simulink model "simulador2017b_v1"  (R2017b)
settings: Solver=FixedStepAuto  StartTime=0.0  StopTime=10  FixedStep=ST  RelTol=1e-3
undefined symbols (not defined in the file or in its folder): b, c_bar, CD_deltae, CDp, CDq, CL0, Cl0, CL_alpha, Cl_beta, Cl_da, CL_deltae, Cl_dr, Cl_p, Cl_r, CLq, Cm0, Cm_alpha, Cm_de, Cm_df, Cm_q, Cn0, Cn_beta, Cn_da, Cn_dr, Cn_p, Cn_r, Cx_df, Cx_dr, Cy0, Cy_beta, Cy_da, Cy_dr, Cy_p, Cy_r, Cz_df, delta_max, Earth, F, i0, k1, k2, KQ, Kv, Light, M, mass, maxRPM, MIL, N, R, ST, T, V, Vmax, Vw_unif, WGS84
libraries: aerolibwind2 x3, aerolibtransform2 x2, aerolibasang x2, aerolibanimutils x1, aerolibfltsims x1, simulink_extras x1, aerolibatmos2 x1, shared6dof x1, aerolibadyn x1
(part 1 of 2)
settings Model: Creator=rablanco.ext  LastModifiedBy=CC
settings SolverCC: ZeroCrossAlgorithm=Adaptive
settings DebuggingCC: AlgebraicLoopMsg=none

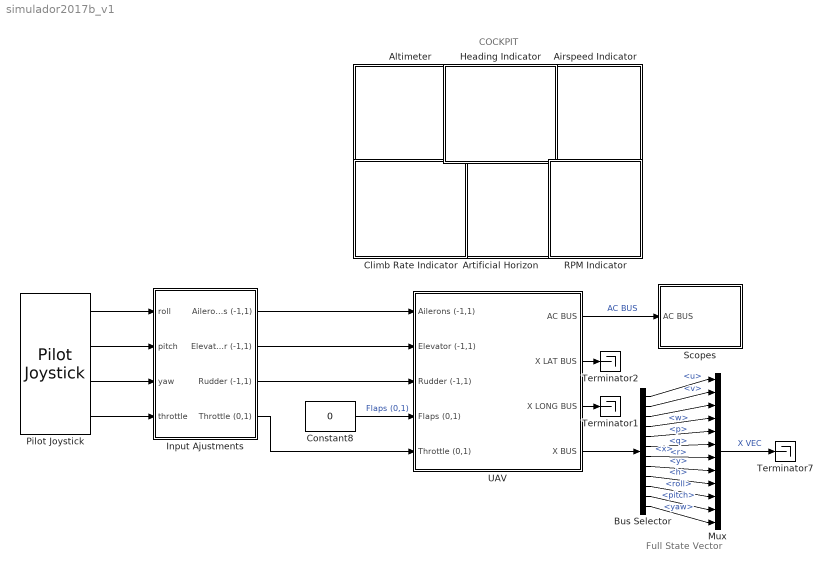
== system simulador2017b_v1 ==
  note: COCKPIT
  note: Full State Vector
  Airspeed Indicator : Subsystem  DialogController=aeroblksHMICreateDDGDialog  IsWebBlock=on  mask(MWDashboardBlock){webBlockId=0719782b-36e5-44f5-ad02-04d1cd166071, webBlockType=airspeedindicator, ShowInLibBrowser=on, ShowInitialText=on, HMISrcModelName=simulador2017b_v1}
      mask prompts: webBlockId "WebBlock Id"; webBlockType "WebBlock Type"; HMISrcModelName "Source Model"
      mask help: Display aircraft airspeed in knots.
      mask Help: asbhmihelp('airspeedindicator')
      mask Display:
      | if strcmp(get_param(bdroot(gcb),'BlockDiagramType'), 'library')
      |  image([(matlabroot) '/toolbox/aeroblks/aeroblks/hmi/icons/AirspeedIndicatorIcon.svg'])
      | end
  Altimeter : Subsystem  DialogController=aeroblksHMICreateDDGDialog  IsWebBlock=on  mask(MWDashboardBlock){webBlockId=d9dc4979-4f2a-46e8-a381-7c2968eac84c, webBlockType=altimeter, ShowInLibBrowser=on, ShowInitialText=on, HMISrcModelName=simulador2017b_v1}
      mask prompts: webBlockId "WebBlock Id"; webBlockType "WebBlock Type"; HMISrcModelName "Source Model"
      mask help: Display aircraft altitude in feet.
      mask Help: asbhmihelp('altimeter')
      mask Display:
      | if strcmp(get_param(bdroot(gcb),'BlockDiagramType'), 'library')
      |  image([(matlabroot) '/toolbox/aeroblks/aeroblks/hmi/icons/AltimeterIcon.svg'])
      | end
  Artificial Horizon : Subsystem  DialogController=aeroblksHMICreateDDGDialog  IsWebBlock=on  mask(MWDashboardBlock){webBlockId=07832adf-b17d-4d9e-ad18-10cd735fd072, webBlockType=artificialhorizon, ShowInLibBrowser=on, ShowInitialText=on, HMISrcModelName=simulador2017b_v1}
      mask prompts: webBlockId "WebBlock Id"; webBlockType "WebBlock Type"; HMISrcModelName "Source Model"
      mask help: Display aircraft attitude relative to horizon. The two signal input vector contains roll and pitch.
      mask Help: asbhmihelp('artificialhorizon')
      mask Display:
      | if strcmp(get_param(bdroot(gcb),'BlockDiagramType'), 'library')
      |  image([(matlabroot) '/toolbox/aeroblks/aeroblks/hmi/icons/ArtificialHorizonIcon.svg'])
      | end
  Bus Selector : BusSelector  OutputSignals=u,v,w,p,q,r,x,y,h,roll,pitch,yaw
  Climb Rate Indicator : Subsystem  DialogController=aeroblksHMICreateDDGDialog  IsWebBlock=on  mask(MWDashboardBlock){webBlockId=6f82ebd9-12ab-4ae3-b879-fc3c75439e10, webBlockType=climbindicator, ShowInLibBrowser=on, ShowInitialText=on, HMISrcModelName=simulador2017b_v1}
      mask prompts: webBlockId "WebBlock Id"; webBlockType "WebBlock Type"; HMISrcModelName "Source Model"
      mask help: Display aircraft climb rate in ft/min.
      mask Help: asbhmihelp('climbindicator')
      mask Display:
      | if strcmp(get_param(bdroot(gcb),'BlockDiagramType'), 'library')
      |  image([(matlabroot) '/toolbox/aeroblks/aeroblks/hmi/icons/ClimbIndicatorIcon.svg'])
      | end
  Constant8 : Constant  Value=0
  Heading Indicator : Subsystem  DialogController=aeroblksHMICreateDDGDialog  IsWebBlock=on  mask(MWDashboardBlock){webBlockId=75353ccd-7314-467c-8fad-26cd782088f3, webBlockType=headingindicator, ShowInLibBrowser=on, ShowInitialText=on, HMISrcModelName=simulador2017b_v1}
      mask prompts: webBlockId "WebBlock Id"; webBlockType "WebBlock Type"; HMISrcModelName "Source Model"
      mask help: Display aircraft heading with respect to North in degrees.
      mask Help: asbhmihelp('headingindicator')
      mask Display:
      | if strcmp(get_param(bdroot(gcb),'BlockDiagramType'), 'library')
      |  image([(matlabroot) '/toolbox/aeroblks/aeroblks/hmi/icons/HeadingIndicatorIcon.svg'])
      | end
  Input Ajustments : Subsystem
  Mux : Mux  Inputs=12
  "Pilot Joystick " : aerolibanimutils/Pilot Joystick  JoystickID=Joystick1  OutputConfiguration=FourAxis  SampleTime=ST
  RPM Indicator : Subsystem  DialogController=aeroblksHMICreateDDGDialog  IsWebBlock=on  mask(MWDashboardBlock){webBlockId=8c376309-98f9-4b67-9096-3662e58f3d70, webBlockType=rpmindicator, ShowInLibBrowser=on, ShowInitialText=on, HMISrcModelName=simulador2017b_v1}
      mask prompts: webBlockId "WebBlock Id"; webBlockType "WebBlock Type"; HMISrcModelName "Source Model"
      mask help: Display engine revolutions per minute (RPM).
      mask Help: asbhmihelp('rpmindicator')
      mask Display:
      | if strcmp(get_param(bdroot(gcb),'BlockDiagramType'), 'library')
      |  image([(matlabroot) '/toolbox/aeroblks/aeroblks/hmi/icons/RPMIndicatorIcon.svg'])
      | end
  Scopes : Subsystem
  Terminator1 : Terminator
  Terminator2 : Terminator
  Terminator7 : Terminator
  UAV : Subsystem  InitFcn=run('..\config_model.m')  StopFcn=|  mask{eulerInit=[0.0014,-0.023,0], ratesInit=[0.1729,0,-0.0277], VbInit=[53.287,-0.958,-1.1917], XeInit=[0 0 -100]}
      | save simulationData Va beta alpha p_meas q_meas r_meas rho deltaa deltae deltar deltat accX accY accZ;
      | save fullStateData time u v w p q r x y z phi theta psi;
      | aileronValMatrix = [time,ailerons_val];
      | elevatorValMatrix = [time,elevator_val];
      | rudderValMatrix = [time,rudder_val];
      | throttleValMatrix = [time,throttle_val];
      mask DialogControl DescGroupVar Prompt: Fixed-Wing UAV Model - V3 - Simplified Version
      mask DialogControl DescTextVar Prompt: This version of the model uses a simplified propulsive model based on the Momentum Theory (Froude Ideal Theory or Disk Actuator Theory) and a simplified polar curve that consists of a linear relationship between the drag coefficient CD and the AOA.
      mask DialogControl Control2 Prompt: INITIAL CONDITIONS for the state integrators: X0.
      mask DialogControl Control4 Prompt: Euler Angles
      mask DialogControl Control4_copy_copy Prompt: Angular Rates - Body Axis
      mask DialogControl Control4_copy Prompt: Ground/Inertial Velocity - Body Axis
      mask DialogControl Control4_copy_copy_copy Prompt: Position (Flat-Earth Model) - NED Axis
  wires:
  UAV/4(X BUS) -> Bus Selector/1
  UAV/2(X LAT BUS) -> Terminator2/1
  UAV/3(X LONG BUS) -> Terminator1/1
  Bus Selector/3 -> Mux/3  "<w>"
  Bus Selector/4 -> Mux/4  "<p>"
  Bus Selector/5 -> Mux/5  "<q>"
  Bus Selector/6 -> Mux/6  "<r>"
  Bus Selector/9 -> Mux/9  "<h>"
  Bus Selector/1 -> Mux/1  "<u>"
  Bus Selector/2 -> Mux/2  "<v>"
  Mux/1 -> Terminator7/1  "X VEC"
  Bus Selector/10 -> Mux/10  "<roll>"
  Bus Selector/11 -> Mux/11  "<pitch>"
  Bus Selector/12 -> Mux/12  "<yaw>"
  Bus Selector/8 -> Mux/8  "<y>"
  Bus Selector/7 -> Mux/7  "<x>"
  UAV/1(AC BUS) -> Scopes/1(AC BUS)  "AC BUS"
  Input Ajustments/4(Throttle (0,1)) -> UAV/5(Throttle (0,1))
  "Pilot Joystick "/1 -> Input Ajustments/1(roll)
  Input Ajustments/3(Rudder (-1,1)) -> UAV/3(Rudder (-1,1))
  "Pilot Joystick "/2 -> Input Ajustments/2(pitch)
  "Pilot Joystick "/3 -> Input Ajustments/3(yaw)
  Input Ajustments/1(Ailerons (-1,1)) -> UAV/1(Ailerons (-1,1))
  Constant8/1 -> UAV/4(Flaps (0,1))  "Flaps (0,1)"
  Input Ajustments/2(Elevator (-1,1)) -> UAV/2(Elevator (-1,1))
  "Pilot Joystick "/4 -> Input Ajustments/4(throttle)

== system simulador2017b_v1/Airspeed Indicator ==

== system simulador2017b_v1/Altimeter ==

== system simulador2017b_v1/Artificial Horizon ==

== system simulador2017b_v1/Climb Rate Indicator ==

== system simulador2017b_v1/Heading Indicator ==

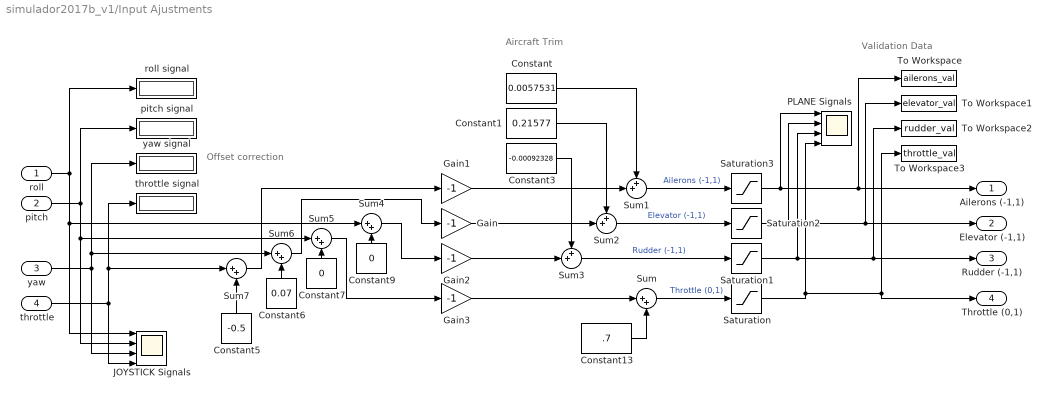
== system simulador2017b_v1/Input Ajustments ==
  note: Validation Data
  note: Aircraft Trim
  note: Offset correction
  roll : Inport
  pitch : Inport  Port=2
  yaw : Inport  Port=3
  throttle : Inport  Port=4
  Constant : Constant  Value=0.0057531
  Constant1 : Constant  Value=0.21577
  Constant13 : Constant  Value=.7
  Constant3 : Constant  Value=-0.00092328
  Constant5 : Constant  Value=-0.5
  Constant6 : Constant  Value=0.07
  Constant7 : Constant  Value=0
  Constant9 : Constant  Value=0
  Gain{,1..3} (4 alike) : Gain  Gain=-1
  "JOYSTICK Signals " : Scope  NumInputPorts=4
  "PLANE Signals " : Scope  NumInputPorts=4
  Saturation : Saturate  UpperLimit=1  LowerLimit=0
  Saturation1 : Saturate  UpperLimit=1  LowerLimit=-1
  Saturation2 : Saturate  UpperLimit=1  LowerLimit=-1
  Saturation3 : Saturate  UpperLimit=1  LowerLimit=-1
  Sum{,4..7} (5 alike) : Sum  Inputs=|++
  Sum1 : Sum  Inputs=++|
  Sum2 : Sum  Inputs=++|
  Sum3 : Sum  Inputs=++|
  To Workspace : ToWorkspace  VariableName=ailerons_val  SampleTime=-1
  To Workspace1 : ToWorkspace  VariableName=elevator_val  SampleTime=-1
  To Workspace2 : ToWorkspace  VariableName=rudder_val  SampleTime=-1
  To Workspace3 : ToWorkspace  VariableName=throttle_val  SampleTime=-1
  pitch signal : Display
  roll signal : Display
  throttle signal : Display
  yaw signal : Display
  Ailerons (-1,1) : Outport
  Elevator (-1,1) : Outport  Port=2
  Rudder (-1,1) : Outport  Port=3
  Throttle (0,1) : Outport  Port=4
  wires:
  pitch/1 -> "JOYSTICK Signals "/2, Sum5/1, pitch signal/1
  Constant1/1 -> Sum2/1
  throttle/1 -> Sum7/1, throttle signal/1, "JOYSTICK Signals "/4
  Sum/1 -> Saturation/1  "Throttle (0,1)"
  Constant/1 -> Sum1/1
  Constant7/1 -> Sum5/2
  Sum2/1 -> Saturation2/1  "Elevator (-1,1)"
  Gain2/1 -> Sum3/2
  roll/1 -> roll signal/1, "JOYSTICK Signals "/1, Sum4/1
  Sum4/1 -> Gain2/1
  Sum1/1 -> Saturation3/1  "Ailerons (-1,1)"
  Constant5/1 -> Sum7/2
  Gain1/1 -> Sum1/2
  Sum6/1 -> Gain/1
  Constant13/1 -> Sum/2
  Constant3/1 -> Sum3/1
  Sum3/1 -> Saturation1/1  "Rudder (-1,1)"
  Gain3/1 -> Sum/1
  yaw/1 -> yaw signal/1, Sum6/1, "JOYSTICK Signals "/3
  Sum7/1 -> Gain1/1
  Constant6/1 -> Sum6/2
  Constant9/1 -> Sum4/2
  Sum5/1 -> Gain3/1
  Gain/1 -> Sum2/2
  Saturation/1 -> "PLANE Signals "/4, Throttle (0,1)/1, To Workspace3/1
  Saturation1/1 -> "PLANE Signals "/3, Rudder (-1,1)/1, To Workspace2/1
  Saturation2/1 -> "PLANE Signals "/2, To Workspace1/1, Elevator (-1,1)/1
  Saturation3/1 -> "PLANE Signals "/1, To Workspace/1, Ailerons (-1,1)/1

== system simulador2017b_v1/RPM Indicator ==

== system simulador2017b_v1/Scopes ==
  AC BUS : Inport
  Attitude Scope : Scope  NumInputPorts=3
  Constant : Constant  Value=0
  Control Scope : Scope  NumInputPorts=5
  Demux : Demux  Outputs=2
  Flat Earth to LLA : aerolibtransform2/Flat Earth to LLA  units=Metric (MKS)  ptype=Earth (WGS84)  F=1/298.257223563  R=6378137  LL0=LatLong0  psi=0
  FlightGear Preconfigured 6DoF Animation : aerolibfltsims/FlightGear Preconfigured 6DoF Animation  xFlightGearVersion=v2017.1  DestinationIpAddress=127.0.0.1  DestinationPort=5502  SampleTime=0.01
      settings: SourceProductName=Aerospace Blockset
  Gain : Gain  Gain=-1
  Lateral Dynamics : Scope
  Longitudinal Dynamics : Scope
  Mux : Mux  Inputs=2
  Mux1 : Mux  Inputs=2
  Mux2 : Mux  Inputs=2
  Position Scope : Scope  NumInputPorts=3
  Propulsion Scope : Scope  NumInputPorts=3
  Selector : Selector  InputPortWidth=3  IndexOptions=Index vector (dialog)  Indices=[3]  OutputSizes=1
  Terminator : Terminator
  Visualization BOX : Subsystem
  wires:
  Visualization BOX/15(u (kph)) -> Propulsion Scope/2
  Visualization BOX/13(Throttle (%)) -> Control Scope/5
  Visualization BOX/8(Height_m) -> Position Scope/3
  Visualization BOX/11(Ailerons (deg)) -> Control Scope/3
  Visualization BOX/3(roll_deg) -> Attitude Scope/1
  AC BUS/1 -> Visualization BOX/1("AC BUS ")
  Visualization BOX/7(East_km) -> Position Scope/2
  Visualization BOX/9(Elevator (deg)) -> Control Scope/1
  Visualization BOX/10(Rudder (deg)) -> Control Scope/2
  Visualization BOX/14(<Thrust>) -> Propulsion Scope/1
  Visualization BOX/16(<RPM>) -> Propulsion Scope/3
  Visualization BOX/12(flaps (deg)) -> Control Scope/4
  Visualization BOX/4(pitch_deg) -> Attitude Scope/2
  Visualization BOX/6(North_km) -> Position Scope/1
  Visualization BOX/5(yaw_deg) -> Attitude Scope/3
  Visualization BOX/17(Longitudinal BUS) -> Longitudinal Dynamics/1
  Visualization BOX/18(Lateral BUS) -> Lateral Dynamics/1
  Mux2/1 -> Mux1/1
  Demux/2 -> Mux2/1
  Demux/1 -> Mux2/2
  Constant/1 -> Flat Earth to LLA/2
  Mux1/1 -> Mux/1
  Visualization BOX/1(Xe) -> Selector/1, Flat Earth to LLA/1
  Visualization BOX/2(<phi theta psi>) -> Mux/2
  Gain/1 -> Mux1/2
  Selector/1 -> Gain/1
  Mux/1 -> FlightGear Preconfigured 6DoF Animation/1
  Flat Earth to LLA/1 -> Demux/1
  Flat Earth to LLA/2 -> Terminator/1

== system simulador2017b_v1/UAV ==
  Ailerons (-1,1) : Inport
  Elevator (-1,1) : Inport  Port=2
  Rudder (-1,1) : Inport  Port=3
  Flaps (0,1) : Inport  Port=4
  Throttle (0,1) : Inport  Port=5
  AC State Creator : Subsystem
  Control BUS Creator : Subsystem
  Environment Model : Subsystem
  Flight Data Recorder (FDR) : Subsystem
  "Platform " : Subsystem
  AC BUS : Outport
  X LAT BUS : Outport  Port=2
  X LONG BUS : Outport  Port=3
  X BUS : Outport  Port=4
  wires:
  Environment Model/1(Environment BUS (ENV BUS)) -> "Platform "/1(ENV BUS)
  Control BUS Creator/1(Control BUS (CTRL BUS)) -> "Platform "/2(CTRL BUS)
  Elevator (-1,1)/1 -> Control BUS Creator/2(Elevator Command (-1,1))
  Flaps (0,1)/1 -> Control BUS Creator/4(Flaps Command (0,1))
  Rudder (-1,1)/1 -> Control BUS Creator/3(Rudder Command (-1,1))
  Ailerons (-1,1)/1 -> Control BUS Creator/1(Ailerons Command (-1,1))
  Throttle (0,1)/1 -> Control BUS Creator/5("Throttle Command (0,1) ")
  "Platform "/1(AC BUS) -> Flight Data Recorder (FDR)/1(AC BUS), Environment Model/1(AC BUS), AC BUS/1, AC State Creator/1(AC BUS)
  AC State Creator/1(X BUS) -> X BUS/1
  AC State Creator/2(X LONG BUS) -> X LONG BUS/1
  AC State Creator/3(X LAT BUS) -> X LAT BUS/1

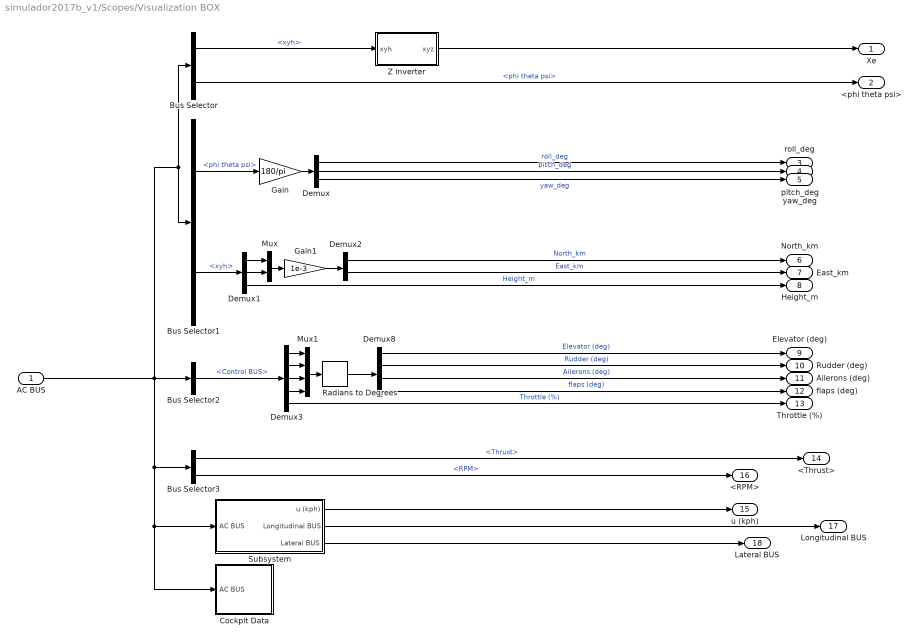
== system simulador2017b_v1/Scopes/Visualization BOX ==
  "AC BUS " : Inport
  Bus Selector : BusSelector  OutputSignals=xyh,phi theta psi
  Bus Selector1 : BusSelector  OutputSignals=phi theta psi,xyh
  Bus Selector2 : BusSelector  OutputSignals=Control BUS
  Bus Selector3 : BusSelector  OutputSignals=Propulsion Data BUS.Thrust,Propulsion Data BUS.RPM
  Cockpit Data : Subsystem
  Demux : Demux  Outputs=3
  Demux1 : Demux  Outputs=3
  Demux2 : Demux  Outputs=2
  Demux3 : Demux  Outputs=5
  Demux8 : Demux
  Gain : Gain  Gain=180/pi
  Gain1 : Gain  Gain=1e-3
  Mux : Mux  Inputs=2
  Mux1 : Mux
  Radians to Degrees : simulink_extras/Transformations/Radians to Degrees
  Subsystem : Subsystem
  Z inverter : Subsystem
  Xe : Outport
  <phi theta psi> : Outport  Port=2
  roll_deg : Outport  Port=3
  pitch_deg : Outport  Port=4
  yaw_deg : Outport  Port=5
  North_km : Outport  Port=6
  East_km : Outport  Port=7
  Height_m : Outport  Port=8
  Elevator (deg) : Outport  Port=9
  Rudder (deg) : Outport  Port=10
  Ailerons (deg) : Outport  Port=11
  flaps (deg) : Outport  Port=12
  Throttle (%) : Outport  Port=13
  <Thrust> : Outport  Port=14
  u (kph) : Outport  Port=15
  <RPM> : Outport  Port=16
  Longitudinal BUS : Outport  Port=17
  Lateral BUS : Outport  Port=18
  wires:
  Subsystem/2(Longitudinal BUS) -> Longitudinal BUS/1
  Subsystem/3(Lateral BUS) -> Lateral BUS/1
  Subsystem/1(u (kph)) -> u (kph)/1
  Bus Selector1/2 -> Demux1/1  "<xyh>"
  Demux1/3 -> Height_m/1  "Height_m"
  Demux/3 -> yaw_deg/1  "yaw_deg"
  Gain/1 -> Demux/1
  Demux/1 -> roll_deg/1  "roll_deg"
  Demux1/2 -> Mux/2
  Bus Selector1/1 -> Gain/1  "<phi theta psi>"
  Demux2/2 -> East_km/1  "East_km"
  Bus Selector2/1 -> Demux3/1  "<Control BUS>"
  Gain1/1 -> Demux2/1
  Bus Selector/2 -> <phi theta psi>/1  "<phi theta psi>"
  Bus Selector/1 -> Z inverter/1(xyh)  "<xyh>"
  Demux1/1 -> Mux/1
  "AC BUS "/1 -> Bus Selector3/1, Subsystem/1(AC BUS), Cockpit Data/1(AC BUS), Bus Selector2/1, Bus Selector/1, Bus Selector1/1
  Demux2/1 -> North_km/1  "North_km"
  Demux/2 -> pitch_deg/1  "pitch_deg"
  Mux/1 -> Gain1/1
  Demux3/4 -> Mux1/4
  Mux1/1 -> Radians to Degrees/1
  Demux3/5 -> Throttle (%)/1  "Throttle (%)"
  Bus Selector3/1 -> <Thrust>/1  "<Thrust>"
  Bus Selector3/2 -> <RPM>/1  "<RPM>"
  Radians to Degrees/1 -> Demux8/1
  Demux3/3 -> Mux1/3
  Demux3/1 -> Mux1/1
  Demux3/2 -> Mux1/2
  Z inverter/1(xyz) -> Xe/1
  Demux8/1 -> Elevator (deg)/1  "Elevator (deg)"
  Demux8/4 -> flaps (deg)/1  "flaps (deg)"
  Demux8/3 -> Ailerons (deg)/1  "Ailerons (deg)"
  Demux8/2 -> Rudder (deg)/1  "Rudder (deg)"

== system simulador2017b_v1/UAV/AC State Creator ==
  AC BUS : Inport
  Bus Creator : BusCreator  Inputs=12
  Bus Creator1 : BusCreator  Inputs=7
  Bus Creator2 : BusCreator  Inputs=7
  Bus Selector : BusSelector  OutputSignals=Air Data BUS.alpha,uvw,pqr,xyh,phi theta psi,Air Data BUS.beta
  Demux{,1..3} (4 alike) : Demux  Outputs=3
  X BUS : Outport
  X LONG BUS : Outport  Port=2
  X LAT BUS : Outport  Port=3
  wires:
  Demux2/2 -> Bus Creator1/4, Bus Creator/8  "y"
  Bus Creator/1 -> X BUS/1  "X BUS"
  Demux/2 -> Bus Creator1/1, Bus Creator/2  "v"
  Demux3/3 -> Bus Creator/12, Bus Creator1/6  "yaw"
  Demux3/2 -> Bus Creator2/6, Bus Creator/11  "pitch"
  Demux1/1 -> Bus Creator1/2, Bus Creator/4  "p"
  Demux1/3 -> Bus Creator1/3, Bus Creator/6  "r"
  AC BUS/1 -> Bus Selector/1  "AC BUS"
  Bus Selector/5 -> Demux3/1  "<phi theta psi>"
  Bus Selector/2 -> Demux/1  "<uvw>"
  Bus Selector/3 -> Demux1/1  "<pqr>"
  Demux3/1 -> Bus Creator1/5, Bus Creator/10  "roll"
  Bus Selector/4 -> Demux2/1  "<xyh>"
  Demux/1 -> Bus Creator2/1, Bus Creator/1  "u"
  Demux1/2 -> Bus Creator/5, Bus Creator2/3  "q"
  Demux2/1 -> Bus Creator2/4, Bus Creator/7  "x"
  Demux2/3 -> Bus Creator2/5, Bus Creator/9  "h"
  Demux/3 -> Bus Creator2/2, Bus Creator/3  "w"
  Bus Creator2/1 -> X LONG BUS/1  "X LONG BUS"
  Bus Creator1/1 -> X LAT BUS/1  "X LAT BUS"
  Bus Selector/1 -> Bus Creator2/7  "<alpha>"
  Bus Selector/6 -> Bus Creator1/7  "<beta>"

== system simulador2017b_v1/UAV/Control BUS Creator ==
  Ailerons Command (-1,1) : Inport
  Elevator Command (-1,1) : Inport  Port=2
  Rudder Command (-1,1) : Inport  Port=3
  Flaps Command (0,1) : Inport  Port=4
  "Throttle Command (0,1) " : Inport  Port=5
  Bus Creator1 : BusCreator  Inputs=5
  Demux : Demux
  Mux : Mux
  Posible Flap positions in % of the delta_max : Lookup_n-D  NumberOfTableDimensions=1  LookupTableObject=''  BreakpointsForDimension1=[0:3]  Table=[0 .2 .6 1]  SaturateOnIntegerOverflow=on  InputSameDT=on
  Rate Limiter : RateLimiter  RisingSlewLimit=0.5  FallingSlewLimit=-0.5
  Saturation : Saturate  UpperLimit=delta_max  LowerLimit=-delta_max
  Saturation1 : Saturate  UpperLimit=1  LowerLimit=0
  Saturation2 : Saturate  UpperLimit=1  LowerLimit=0
  max deflection (rad) : Gain  Gain=delta_max
  Control BUS (CTRL BUS) : Outport
  wires:
  Demux/2 -> Bus Creator1/2  "deltae"
  Demux/1 -> Bus Creator1/1  "deltaa"
  Demux/4 -> Bus Creator1/4  "deltaf"
  Demux/3 -> Bus Creator1/3  "deltar"
  Bus Creator1/1 -> Control BUS (CTRL BUS)/1  "Control BUS"
  Mux/1 -> max deflection (rad)/1
  Rudder Command (-1,1)/1 -> Mux/3
  Ailerons Command (-1,1)/1 -> Mux/1
  max deflection (rad)/1 -> Saturation/1
  Elevator Command (-1,1)/1 -> Mux/2
  Rate Limiter/1 -> Posible Flap positions in % of the delta_max/1
  "Throttle Command (0,1) "/1 -> Saturation1/1  "deltat"
  Saturation/1 -> Demux/1
  Saturation1/1 -> Bus Creator1/5  "deltat"
  Posible Flap positions in % of the delta_max/1 -> Mux/4
  Flaps Command (0,1)/1 -> Saturation2/1
  Saturation2/1 -> Rate Limiter/1

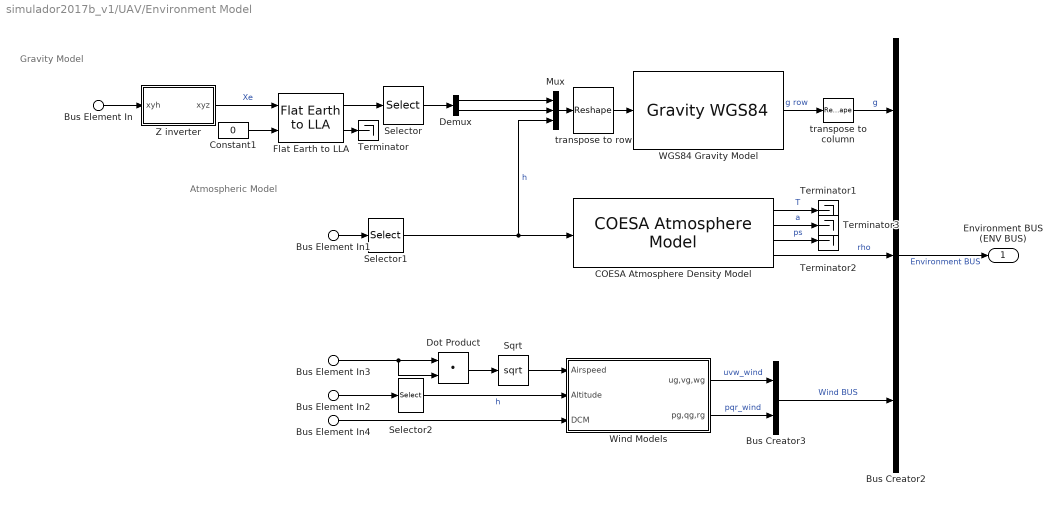
== system simulador2017b_v1/UAV/Environment Model ==
  note: Gravity Model
  note: Atmospheric Model
  Bus Element In : Inport  PortName=AC BUS  Element=xyh
  Bus Element In1 : Inport  PortName=AC BUS  Element=xyh
  Bus Element In2 : Inport  PortName=AC BUS  Element=xyh
  Bus Element In4 : Inport  PortName=AC BUS  Element=DCMbe
  Bus Element In3 : Inport  PortName=AC BUS  Element="xdot  ydot  zdot"
  Bus Creator2 : BusCreator  Inputs=3
  Bus Creator3 : BusCreator  Inputs=2
  COESA Atmosphere Density Model : aerolibatmos2/COESA Atmosphere Model  units=Metric (MKS)  spec=1976 COESA-extended U.S. Standard Atmosphere  model=Profile  profile_var=High temperature  profile_percent=1%  profile_alt=5 km (16404 ft)  envelope_var=High temperature  envelope_percent=1%  action=Warning
  Constant1 : Constant  Value=0
  Demux : Demux  Outputs=2
  Dot Product : DotProduct  InputSameDT=on  OutDataTypeStr=Inherit: Inherit via internal rule
  "Flat Earth to LLA " : aerolibtransform2/Flat Earth to LLA  units=Metric (MKS)  ptype=Earth (WGS84)  F=1/298.257223563  R=6378137  LL0=LatLong0  psi=0
  Mux : Mux  Inputs=3
  Selector : Selector  IndexMode=Zero-based  InputPortWidth=2  IndexOptions=Index vector (dialog)  Indices=[1 0]  OutputSizes=1
  Selector1 : Selector  IndexMode=Zero-based  InputPortWidth=3  IndexOptions=Index vector (dialog)  Indices=2  OutputSizes=1
  Selector2 : Selector  IndexMode=Zero-based  InputPortWidth=3  IndexOptions=Index vector (dialog)  Indices=2  OutputSizes=1
  Sqrt : Sqrt  SaturateOnIntegerOverflow=on
  Terminator{,1..3} (4 alike) : Terminator
  "WGS84 Gravity Model " : GravityWGS84  action=None
  Wind Models : Subsystem
  Z inverter : Subsystem
  transpose to column : Reshape  OutputDimensionality=Column vector (2-D)
  transpose to row : Reshape  OutputDimensionality=Row vector (2-D)
  Environment BUS (ENV BUS) : Outport
  wires:
  Bus Creator2/1 -> Environment BUS (ENV BUS)/1  "Environment BUS"
  Bus Creator3/1 -> Bus Creator2/3  "Wind BUS"
  Demux/1 -> Mux/1
  "Flat Earth to LLA "/2 -> Terminator/1
  Demux/2 -> Mux/2
  "WGS84 Gravity Model "/1 -> transpose to column/1  "g row"
  COESA Atmosphere Density Model/3 -> Terminator2/1  "ps"
  COESA Atmosphere Density Model/1 -> Terminator1/1  "T"
  Bus Element In1/1 -> Selector1/1
  transpose to row/1 -> "WGS84 Gravity Model "/1
  Mux/1 -> transpose to row/1
  Bus Element In4/1 -> Wind Models/3(DCM)
  COESA Atmosphere Density Model/4 -> Bus Creator2/2  "rho"
  Selector2/1 -> Wind Models/2(Altitude)  "h"
  Bus Element In2/1 -> Selector2/1
  COESA Atmosphere Density Model/2 -> Terminator3/1  "a"
  Selector/1 -> Demux/1
  Constant1/1 -> "Flat Earth to LLA "/2
  "Flat Earth to LLA "/1 -> Selector/1
  Bus Element In/1 -> Z inverter/1(xyh)
  Z inverter/1(xyz) -> "Flat Earth to LLA "/1  "Xe"
  Wind Models/1(ug,vg,wg) -> Bus Creator3/1  "uvw_wind"
  Wind Models/2(pg,qg,rg) -> Bus Creator3/2  "pqr_wind"
  Selector1/1 -> COESA Atmosphere Density Model/1, Mux/3  "h"
  transpose to column/1 -> Bus Creator2/1  "g"
  Bus Element In3/1 -> Dot Product/2, Dot Product/1
  Dot Product/1 -> Sqrt/1
  Sqrt/1 -> Wind Models/1(Airspeed)

== system simulador2017b_v1/UAV/Flight Data Recorder (FDR) ==
  note: - accX
  note: OUTPUTS TO WORKSPACE
  note: - accY
  note: - accZ
  note: - p_meas
  note: - r_meas
  note: - q_meas
  AC BUS : Inport
  Clock : Clock
  IMU Sensor Recorder : Subsystem
  Other Sensors Recorder : Subsystem
  Real State Recorder : Subsystem
  To Workspace10 : ToWorkspace  VariableName=time  SampleTime=-1
  wires:
  Clock/1 -> To Workspace10/1
  AC BUS/1 -> Real State Recorder/1(AC BUS), IMU Sensor Recorder/1(AC BUS), Other Sensors Recorder/1(AC BUS)

== system simulador2017b_v1/UAV/Platform  ==
  ENV BUS : Inport
  CTRL BUS : Inport  Port=2
  Air Data System : Subsystem
  Aircraft Mechanics : Subsystem
  AC BUS : Outport
  wires:
  Air Data System/1(Air Data BUS (AD BUS)) -> Aircraft Mechanics/1(AD BUS)
  ENV BUS/1 -> Air Data System/2(ENV BUS), Aircraft Mechanics/3(ENV BUS)
  Aircraft Mechanics/1(AC BUS) -> Air Data System/1(AC BUS), AC BUS/1
  CTRL BUS/1 -> Aircraft Mechanics/2(CTRL BUS)

== system simulador2017b_v1/Scopes/Visualization BOX/Cockpit Data ==
  AC BUS : Inport
  Bus Selector1 : BusSelector  OutputSignals=uvw,hdot,xyh,phi theta psi,Propulsion Data BUS.RPM
  Demux : Demux  Outputs=3
  Demux1 : Demux  Outputs=3
  Gain : Gain  Gain=3.28084
  Gain1 : Gain  Gain=3.28084*60
  Gain2 : Gain  Gain=180/pi
  Gain3 : Gain  Gain=(1/maxRPM)*100
  MATLAB Function : MATLAB Function  TreatAsAtomicUnit=on
  Mux : Mux  Inputs=2
  Terminator{,1..7} (8 alike) : Terminator
  wires:
  Demux1/3 -> Terminator6/1  "heading_deg"
  Mux/1 -> Terminator5/1  "roll;pitch"
  Bus Selector1/1 -> MATLAB Function/1(uvw)  "<uvw>"
  MATLAB Function/1(airspeed) -> Terminator/1  "airspeed_knots"
  Gain2/1 -> Demux1/1
  Demux/3 -> Gain/1
  Demux/1 -> Terminator1/1
  Gain1/1 -> Terminator4/1  "hdot_ftmin"
  Demux/2 -> Terminator2/1
  Gain/1 -> Terminator3/1  "h_ft"
  Bus Selector1/2 -> Gain1/1  "<hdot>"
  Demux1/1 -> Mux/1
  Bus Selector1/4 -> Gain2/1  "<phi theta psi>"
  Bus Selector1/3 -> Demux/1  "<xyh>"
  Demux1/2 -> Mux/2
  AC BUS/1 -> Bus Selector1/1
  Bus Selector1/5 -> Gain3/1  "<RPM>"
  Gain3/1 -> Terminator7/1  "RPM/1000"

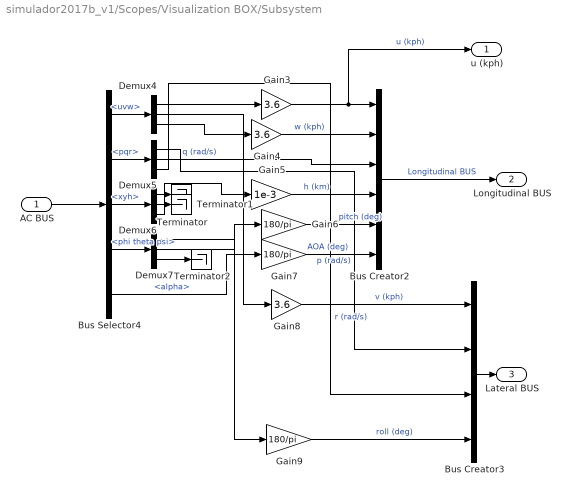
== system simulador2017b_v1/Scopes/Visualization BOX/Subsystem ==
  AC BUS : Inport
  Bus Creator2 : BusCreator  Inputs=6
  Bus Creator3 : BusCreator  Inputs=4
  Bus Selector4 : BusSelector  OutputSignals=uvw,pqr,xyh,phi theta psi,Air Data BUS.alpha
  Demux{4..7} (4 alike) : Demux  Outputs=3
  Gain3 : Gain  Gain=3.6
  Gain4 : Gain  Gain=3.6
  Gain5 : Gain  Gain=1e-3
  Gain6 : Gain  Gain=180/pi
  Gain7 : Gain  Gain=180/pi
  Gain8 : Gain  Gain=3.6
  Gain9 : Gain  Gain=180/pi
  Terminator : Terminator
  Terminator1 : Terminator
  Terminator2 : Terminator
  u (kph) : Outport
  Longitudinal BUS : Outport  Port=2
  Lateral BUS : Outport  Port=3
  wires:
  AC BUS/1 -> Bus Selector4/1
  Demux6/3 -> Gain5/1
  Gain7/1 -> Bus Creator2/6  "AOA (deg)"
  Gain5/1 -> Bus Creator2/4  "h (km)"
  Gain6/1 -> Bus Creator2/5  "pitch (deg)"
  Bus Creator2/1 -> Longitudinal BUS/1  "Longitudinal BUS"
  Bus Creator3/1 -> Lateral BUS/1
  Demux4/2 -> Gain8/1
  Bus Selector4/3 -> Demux6/1  "<xyh>"
  Gain4/1 -> Bus Creator2/2  "w (kph)"
  Bus Selector4/4 -> Demux7/1  "<phi theta psi>"
  Gain8/1 -> Bus Creator3/1  "v (kph)"
  Bus Selector4/5 -> Gain7/1  "<alpha>"
  Demux4/1 -> Gain3/1
  Bus Selector4/2 -> Demux5/1  "<pqr>"
  Bus Selector4/1 -> Demux4/1  "<uvw>"
  Demux5/2 -> Bus Creator2/3  "q (rad/s)"
  Demux7/2 -> Gain6/1
  Gain3/1 -> u (kph)/1, Bus Creator2/1  "u (kph)"
  Demux4/3 -> Gain4/1
  Demux7/3 -> Terminator2/1
  Demux6/2 -> Terminator1/1
  Demux6/1 -> Terminator/1
  Demux7/1 -> Gain9/1
  Demux5/3 -> Bus Creator3/3  "r (rad/s)"
  Demux5/1 -> Bus Creator3/2  "p (rad/s)"
  Gain9/1 -> Bus Creator3/4  "roll (deg)"

== system simulador2017b_v1/Scopes/Visualization BOX/Z inverter ==
  xyh : Inport
  Demux3 : Demux  Outputs=3
  Gain2 : Gain  Gain=-1
  Mux1 : Mux  Inputs=3
  xyz : Outport
  wires:
  Demux3/1 -> Mux1/1
  Gain2/1 -> Mux1/3
  Demux3/3 -> Gain2/1
  Mux1/1 -> xyz/1
  Demux3/2 -> Mux1/2
  xyh/1 -> Demux3/1

== system simulador2017b_v1/UAV/Environment Model/Wind Models ==
  note: Describes how the wind changes speed and/or direction with position (in this case with height)
      | It can be vertical or horizontal.
  note: Describes how the random wind turbulance based on the Dryden Model, that passes white noise through LTI filters with rational terms
  note: Creates custom wind gusts, at any selected time
  Airspeed : Inport  Unit=m/s
  Altitude : Inport  Port=2  Unit=meter
  DCM : Inport  Port=3
  Constant : Constant  Value=Vw_unif
  "DCM " : InportShadow  Port=3
  "Discrete Wind Gust Model " : aerolibwind2/Discrete Wind Gust Model  units=Metric (MKS)  Gx=off  Gy=off  Gz=off  t_0=20  d_m=[120 120 80]  v_m=[3.5 3.5 3.0]
      settings: SourceProductName=Aerospace Blockset
  Dryden Wind Turbulence Model (Continuous (+q -r)) : aerolibwind2/Dryden Wind Turbulence Model  (Continuous (+q -r))  units=Metric (MKS)  spec=MIL-F-8785C  model=Continuous Dryden (+q -r)  W20=5  Wdeg=0  TurbProb=10^-2 - Light  L_high=533.4  Wingspan=4  ts=0.1  Seed=[23341 23342 23343 23344]  T_on=off
      settings: SourceProductName=Aerospace Blockset
  Matrix Multiply : Product  Multiplication=Matrix(*)
  Sum : Sum  Inputs=++++  SaturateOnIntegerOverflow=on  InputSameDT=on  OutDataTypeStr=Inherit: Same as first input
  "Wind Shear Model " : aerolibwind2/Wind Shear Model  units=Metric (MKS)  phase=Category C - Terminal Flight Phase  W_20=0  Wdeg=0
      settings: SourceProductName=Aerospace Blockset
  ug,vg,wg : Outport  Unit=m/s
  pg,qg,rg : Outport  Port=2  Unit=rad/second
  wires:
  "DCM "/1 -> Matrix Multiply/1, Dryden Wind Turbulence Model (Continuous (+q -r))/3  "DCM"
  "Wind Shear Model "/1 -> Sum/1  "Wind Shear Body Axis"
  Dryden Wind Turbulence Model (Continuous (+q -r))/1 -> Sum/2  "Random Gust Body Axis"
  "Discrete Wind Gust Model "/1 -> Sum/3  "Controlled Gust Body Axis"
  Sum/1 -> ug,vg,wg/1
  DCM/1 -> "Wind Shear Model "/2  "DCM"
  Airspeed/1 -> Dryden Wind Turbulence Model (Continuous (+q -r))/2, "Discrete Wind Gust Model "/1
  Dryden Wind Turbulence Model (Continuous (+q -r))/2 -> pg,qg,rg/1
  Altitude/1 -> Dryden Wind Turbulence Model (Continuous (+q -r))/1, "Wind Shear Model "/1
  Matrix Multiply/1 -> Sum/4  "Uniform Wind Body Axis"
  Constant/1 -> Matrix Multiply/2  "Uniform Wind NED Axis"

== system simulador2017b_v1/UAV/Environment Model/Z inverter ==
  xyh : Inport
  Demux3 : Demux  Outputs=3
  Gain2 : Gain  Gain=-1
  Mux1 : Mux  Inputs=3
  xyz : Outport
  wires:
  Demux3/1 -> Mux1/1
  Gain2/1 -> Mux1/3
  Demux3/3 -> Gain2/1
  Mux1/1 -> xyz/1
  Demux3/2 -> Mux1/2
  xyh/1 -> Demux3/1

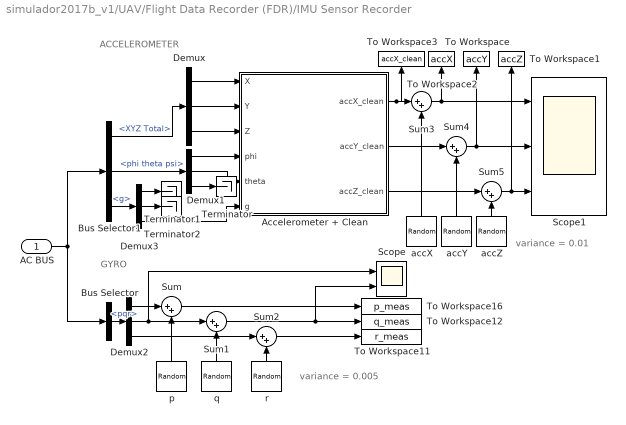
== system simulador2017b_v1/UAV/Flight Data Recorder (FDR)/IMU Sensor Recorder ==
  note: variance = 0.01
  note: GYRO
  note: ACCELEROMETER
  note: variance = 0.005
  AC BUS : Inport
  Accelerometer + Clean : MATLAB Function  TreatAsAtomicUnit=on
  Bus Selector : BusSelector  OutputSignals=pqr
  Bus Selector1 : BusSelector  OutputSignals=XYZ Total,phi theta psi,Environment BUS.g
  Demux{,1..3} (4 alike) : Demux  Outputs=3
  Scope : Scope  NumInputPorts=2
  Scope1 : Scope  NumInputPorts=3
  Sum{,1..5} (6 alike) : Sum  Inputs=|++
  Terminator : Terminator
  Terminator1 : Terminator
  Terminator2 : Terminator
  To Workspace : ToWorkspace  VariableName=accY  SampleTime=-1
  To Workspace1 : ToWorkspace  VariableName=accZ  SampleTime=-1
  To Workspace11 : ToWorkspace  VariableName=r_meas  SampleTime=-1
  To Workspace12 : ToWorkspace  VariableName=q_meas  SampleTime=-1
  To Workspace16 : ToWorkspace  VariableName=p_meas  SampleTime=-1
  To Workspace2 : ToWorkspace  VariableName=accX  SampleTime=-1
  To Workspace3 : ToWorkspace  VariableName=accX_clean  SampleTime=-1
  accX : RandomNumber  Variance=0.16^2  SampleTime=ST
  accY : RandomNumber  Variance=0.16^2  SampleTime=ST
  accZ : RandomNumber  Variance=0.16^2  SampleTime=ST
  p : RandomNumber  Variance=1.2182398178920420446927361564051e-5  SampleTime=ST
  q : RandomNumber  Variance=1.2182398178920420446927361564051e-5  SampleTime=ST
  r : RandomNumber  Variance=1.2182398178920420446927361564051e-5  SampleTime=ST
  wires:
  Demux2/2 -> Sum1/1, Scope/1
  Demux2/1 -> Sum/1
  Demux2/3 -> Sum2/1
  Sum1/1 -> To Workspace12/1, Scope/2
  Sum2/1 -> To Workspace11/1
  Sum/1 -> To Workspace16/1
  Bus Selector/1 -> Demux2/1  "<pqr>"
  AC BUS/1 -> Bus Selector/1, Bus Selector1/1
  Accelerometer + Clean/3(accZ_clean) -> Sum5/1
  Accelerometer + Clean/2(accY_clean) -> Sum4/1
  Bus Selector1/2 -> Demux1/1  "<phi theta psi>"
  Demux/2 -> Accelerometer + Clean/2(Y)
  Demux1/2 -> Accelerometer + Clean/5(theta)
  Demux1/1 -> Accelerometer + Clean/4(phi)
  Demux1/3 -> Terminator/1
  Demux/3 -> Accelerometer + Clean/3(Z)
  Demux/1 -> Accelerometer + Clean/1(X)
  Bus Selector1/1 -> Demux/1  "<XYZ Total>"
  q/1 -> Sum1/2
  r/1 -> Sum2/2
  p/1 -> Sum/2
  Bus Selector1/3 -> Demux3/1  "<g>"
  Demux3/1 -> Terminator1/1
  Demux3/2 -> Terminator2/1
  Demux3/3 -> Accelerometer + Clean/6(g)
  accX/1 -> Sum3/2
  accZ/1 -> Sum5/2
  accY/1 -> Sum4/2
  Sum3/1 -> Scope1/1, To Workspace2/1
  Sum4/1 -> Scope1/2, To Workspace/1
  Sum5/1 -> Scope1/3, To Workspace1/1
  Accelerometer + Clean/1(accX_clean) -> Sum3/1, To Workspace3/1

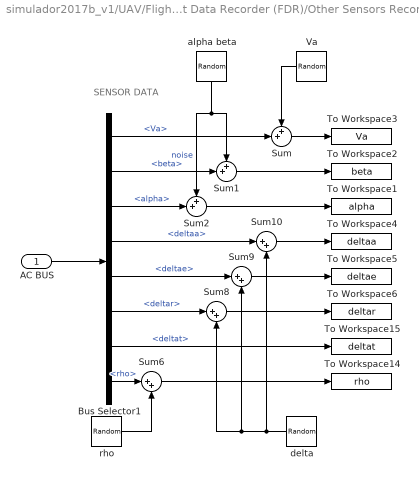
== system simulador2017b_v1/UAV/Flight Data Recorder (FDR)/Other Sensors Recorder ==
  note: SENSOR DATA
  AC BUS : Inport
  Bus Selector1 : BusSelector  OutputSignals=Air Data BUS.Va,Air Data BUS.beta,Air Data BUS.alpha,Control BUS.deltaa,Control BUS.deltae,Control BUS.deltar,Control BUS.deltat,Environment BUS.rho
  Sum : Sum  Inputs=++|
  Sum1 : Sum  Inputs=++|
  Sum{6,8..10} (4 alike) : Sum  Inputs=|++
  Sum2 : Sum  Inputs=++|
  To Workspace1 : ToWorkspace  VariableName=alpha  SampleTime=-1
  To Workspace14 : ToWorkspace  VariableName=rho  SampleTime=-1
  To Workspace15 : ToWorkspace  VariableName=deltat  SampleTime=-1
  To Workspace2 : ToWorkspace  VariableName=beta  SampleTime=-1
  To Workspace3 : ToWorkspace  VariableName=Va  SampleTime=-1
  To Workspace4 : ToWorkspace  VariableName=deltaa  SampleTime=-1
  To Workspace5 : ToWorkspace  VariableName=deltae  SampleTime=-1
  To Workspace6 : ToWorkspace  VariableName=deltar  SampleTime=-1
  Va : RandomNumber  Variance=0.5^2  SampleTime=ST
  alpha beta : RandomNumber  Variance=3.046e-6  SampleTime=ST
  delta : RandomNumber  Variance=3.046e-6  SampleTime=ST
  rho : RandomNumber  Variance=0.001^2  SampleTime=ST
  wires:
  AC BUS/1 -> Bus Selector1/1
  Bus Selector1/1 -> Sum/2  "<Va>"
  Bus Selector1/4 -> Sum10/1  "<deltaa>"
  Bus Selector1/7 -> To Workspace15/1  "<deltat>"
  Bus Selector1/2 -> Sum1/2  "<beta>"
  Bus Selector1/5 -> Sum9/1  "<deltae>"
  Bus Selector1/6 -> Sum8/1  "<deltar>"
  Bus Selector1/3 -> Sum2/2  "<alpha>"
  Bus Selector1/8 -> Sum6/1  "<rho>"
  Sum/1 -> To Workspace3/1
  Sum1/1 -> To Workspace2/1
  Sum2/1 -> To Workspace1/1
  Sum6/1 -> To Workspace14/1
  Sum8/1 -> To Workspace6/1
  Sum9/1 -> To Workspace5/1
  Sum10/1 -> To Workspace4/1
  Va/1 -> Sum/1
  rho/1 -> Sum6/2
  delta/1 -> Sum9/2, Sum8/2, Sum10/2
  alpha beta/1 -> Sum2/1, Sum1/1  "noise"

== system simulador2017b_v1/UAV/Flight Data Recorder (FDR)/Real State Recorder ==
  AC BUS : Inport
  Bus Selector2 : BusSelector  OutputSignals=uvw,pqr,xyh,phi theta psi
  Demux{1..4} (4 alike) : Demux  Outputs=3
  To Workspace11 : ToWorkspace  VariableName=w  SampleTime=-1
  To Workspace12 : ToWorkspace  VariableName=phi  SampleTime=-1
  To Workspace16 : ToWorkspace  VariableName=theta  SampleTime=-1
  To Workspace19 : ToWorkspace  VariableName=v  SampleTime=-1
  To Workspace20 : ToWorkspace  VariableName=u  SampleTime=-1
  To Workspace21 : ToWorkspace  VariableName=x  SampleTime=-1
  To Workspace22 : ToWorkspace  VariableName=y  SampleTime=-1
  To Workspace23 : ToWorkspace  VariableName=z  SampleTime=-1
  To Workspace24 : ToWorkspace  VariableName=r  SampleTime=-1
  To Workspace25 : ToWorkspace  VariableName=q  SampleTime=-1
  To Workspace26 : ToWorkspace  VariableName=p  SampleTime=-1
  To Workspace27 : ToWorkspace  VariableName=psi  SampleTime=-1
  wires:
  Demux2/1 -> To Workspace26/1
  Demux3/1 -> To Workspace12/1
  Bus Selector2/3 -> Demux1/1  "<xyh>"
  Bus Selector2/2 -> Demux2/1  "<pqr>"
  Bus Selector2/1 -> Demux4/1  "<uvw>"
  Bus Selector2/4 -> Demux3/1  "<phi theta psi>"
  Demux3/3 -> To Workspace27/1
  Demux2/3 -> To Workspace24/1
  Demux2/2 -> To Workspace25/1
  Demux3/2 -> To Workspace16/1
  AC BUS/1 -> Bus Selector2/1
  Demux1/1 -> To Workspace21/1
  Demux1/2 -> To Workspace22/1
  Demux1/3 -> To Workspace23/1
  Demux4/3 -> To Workspace11/1
  Demux4/2 -> To Workspace19/1
  Demux4/1 -> To Workspace20/1

== system simulador2017b_v1/UAV/Platform /Air Data System ==
  note: q_bar : dynamic pressure
  Bus Element In3 : Inport  PortName=AC BUS  Element=uvw
  Bus Element In4 : Inport  PortName=AC BUS  Element=pqr
  Bus Element In : Inport  Port=2  PortName=ENV BUS  Element=rho
  Bus Element In1 : Inport  Port=2  PortName=ENV BUS  Element=Wind BUS.uvw_wind
  Bus Element In2 : Inport  Port=2  PortName=ENV BUS  Element=Wind BUS.pqr_wind
  Bus Creator : BusCreator  Inputs=6
  Dynamic Pressure : aerolibasang/Dynamic Pressure
  "Incidence, Sideslip, & Airspeed" : aerolibasang/Incidence, Sideslip, & Airspeed
      settings: SourceProductName=Aerospace Blockset
  Sum2 : Sum  Inputs=++|  SaturateOnIntegerOverflow=on  InputSameDT=on  OutDataTypeStr=Inherit: Same as first input
  Sum4 : Sum  Inputs=+-|  SaturateOnIntegerOverflow=on  InputSameDT=on  OutDataTypeStr=Inherit: Same as first input
  Air Data BUS (AD BUS) : Outport
  wires:
  Dynamic Pressure/1 -> Bus Creator/5  "q_bar"
  "Incidence, Sideslip, & Airspeed"/2 -> Bus Creator/2  "beta"
  "Incidence, Sideslip, & Airspeed"/1 -> Bus Creator/1  "alpha"
  Sum2/1 -> Bus Creator/4  "pqr_tot"
  Bus Element In1/1 -> Sum4/2  "wind - Wind Speed (body axis)"
  Bus Element In/1 -> Dynamic Pressure/2
  Bus Element In2/1 -> Sum2/1
  Bus Element In3/1 -> Sum4/1  "Vg - Ground Speed (body axis)"
  Bus Creator/1 -> Air Data BUS (AD BUS)/1  "Air Data BUS"
  Bus Element In4/1 -> Sum2/2
  Sum4/1 -> "Incidence, Sideslip, & Airspeed"/1, Dynamic Pressure/1, Bus Creator/6  "Va - Aerodynamic Velocity (UAV relative to the air)"
  "Incidence, Sideslip, & Airspeed"/3 -> Bus Creator/3  "Va"

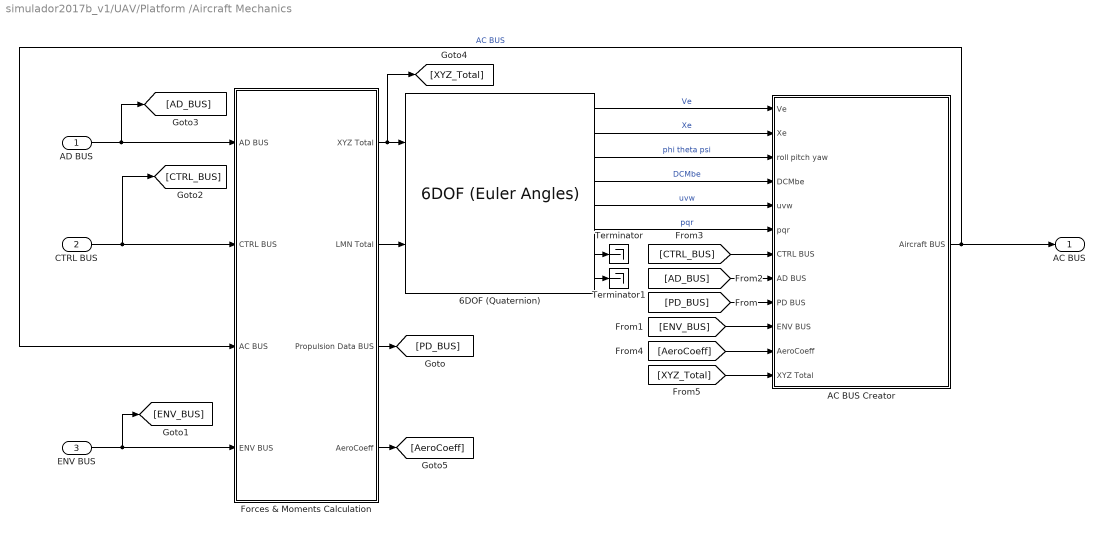
== system simulador2017b_v1/UAV/Platform /Aircraft Mechanics ==
  AD BUS : Inport
  CTRL BUS : Inport  Port=2
  ENV BUS : Inport  Port=3
  6DOF (Quaternion) : shared6dof/6DOF (Euler Angles)  units=Metric (MKS)  mtype=Fixed  rep=Euler Angles  xme_0=XeInit  Vm_0=VbInit  eul_0=eulerInit  pm_0=ratesInit  mass_0=mass  mass_e=0.5  mass_f=2.0  inertia=J  inertia_e=eye(3)  inertia_f=2*eye(3)  k_quat=1.0  vre_flag=on  abi_flag=off
      settings: SourceProductBaseCode=AE
  AC BUS Creator : Subsystem
      mask Display:
      | port_label('input',1,'[(dx/dt) (dy/dt) (dz/dt)]','texmode','on')
      | port_label('input',2,'[x y z]','texmode','on')
      | port_label('input',3,'[\phi \theta \psi]','texmode','on')
      | port_label('input',4,'DCM_e^b','texmode','on')
      | port_label('input',5,'[u v w]','texmode','on')
      | port_label('input',6,'[p q r]','texmode','on')
      | port_label('input',7,'CTRL BUS','texmode','on')
      | port_label('input',8,'AD BUS','texmode','on')
      | port_label('input',9,'PD BUS','texmode','on')
      | port_label('input',10,'ENV BUS','texmode','on')
      | port_label('input',11,'Aero Coeff','texmode','on')
      | port_label('input',12,'XYZ Total','texmode','on')
      | port_label('output',1,'Aircraft BUS (AC BUS)','texmode','on')
  Forces & Moments Calculation : Subsystem
      mask Display:
      | port_label('input',1,'AD BUS','texmode','on')
      | port_label('input',2,'CTRL BUS','texmode','on')
      | port_label('input',4,'ENV BUS','texmode','on')
      | port_label('input',3,'AC BUS','texmode','on')
      | port_label('output',1,'XYZ Total','texmode','on')
      | port_label('output',2,'LMN Total','texmode','on')
      | port_label('output',3,'PD BUS','texmode','on')
      | port_label('output',4,'AeroCoeff','texmode','on')
  Terminator : Terminator
  Terminator1 : Terminator
  AC BUS : Outport
  wires:
  Forces & Moments Calculation/1(XYZ Total) -> [XYZ_Total], 6DOF (Quaternion)/1
  Forces & Moments Calculation/2(LMN Total) -> 6DOF (Quaternion)/2
  CTRL BUS/1 -> [CTRL_BUS], Forces & Moments Calculation/2(CTRL BUS)
  ENV BUS/1 -> Forces & Moments Calculation/4(ENV BUS), [ENV_BUS]
  AC BUS Creator/1(Aircraft BUS) -> AC BUS/1, Forces & Moments Calculation/3(AC BUS)  "AC BUS"
  6DOF (Quaternion)/8 -> Terminator1/1
  6DOF (Quaternion)/7 -> Terminator/1
  Forces & Moments Calculation/3("Propulsion Data BUS ") -> [PD_BUS]
  AD BUS/1 -> [AD_BUS], Forces & Moments Calculation/1(AD BUS)
  [AeroCoeff] -> AC BUS Creator/11(AeroCoeff)
  [CTRL_BUS] -> AC BUS Creator/7(CTRL BUS)
  [AD_BUS] -> AC BUS Creator/8(AD BUS)
  [XYZ_Total] -> AC BUS Creator/12(XYZ Total)
  6DOF (Quaternion)/5 -> AC BUS Creator/5(uvw)  "uvw"
  6DOF (Quaternion)/4 -> AC BUS Creator/4(DCMbe)  "DCMbe"
  6DOF (Quaternion)/3 -> AC BUS Creator/3(roll pitch yaw)  "phi theta psi"
  [PD_BUS] -> AC BUS Creator/9(PD BUS)
  6DOF (Quaternion)/1 -> AC BUS Creator/1(Ve)  "Ve"
  [ENV_BUS] -> AC BUS Creator/10(ENV BUS)
  6DOF (Quaternion)/2 -> AC BUS Creator/2(Xe)  "Xe"
  6DOF (Quaternion)/6 -> AC BUS Creator/6(pqr)  "pqr"
  Forces & Moments Calculation/4(AeroCoeff) -> [AeroCoeff]

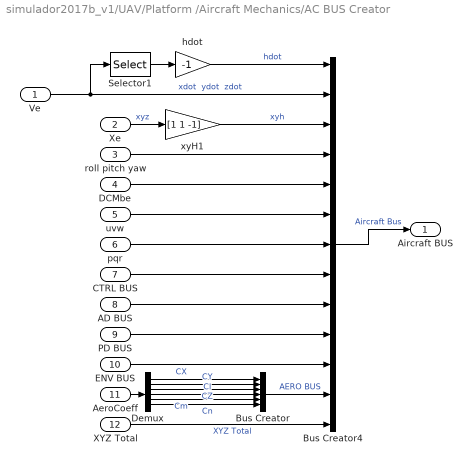
== system simulador2017b_v1/UAV/Platform /Aircraft Mechanics/AC BUS Creator ==
  Ve : Inport
  Xe : Inport  Port=2
  roll pitch yaw : Inport  Port=3
  DCMbe : Inport  Port=4
  uvw : Inport  Port=5
  pqr : Inport  Port=6
  CTRL BUS : Inport  Port=7
  AD BUS : Inport  Port=8
  PD BUS : Inport  Port=9
  ENV BUS : Inport  Port=10
  AeroCoeff : Inport  Port=11
  XYZ Total : Inport  Port=12
  Bus Creator : BusCreator  Inputs=6
  Bus Creator4 : BusCreator  Inputs=13
  Demux : Demux  Outputs=6
  Selector1 : Selector  IndexMode=Zero-based  InputPortWidth=3  IndexOptions=Index vector (dialog)  Indices=2  OutputSizes=1
  hdot : Gain  Gain=-1  SaturateOnIntegerOverflow=on  OutDataTypeStr=Inherit: Same as input  ParamDataTypeStr=Inherit: Same as input
  xyH1 : Gain  Gain=[1 1 -1]  SaturateOnIntegerOverflow=on  OutDataTypeStr=Inherit: Same as input  ParamDataTypeStr=Inherit: Same as input
  Aircraft BUS : Outport
  wires:
  hdot/1 -> Bus Creator4/1  "hdot"
  Ve/1 -> Selector1/1, Bus Creator4/2  "xdot  ydot  zdot"
  pqr/1 -> Bus Creator4/7
  roll pitch yaw/1 -> Bus Creator4/4
  DCMbe/1 -> Bus Creator4/5
  Selector1/1 -> hdot/1
  uvw/1 -> Bus Creator4/6
  xyH1/1 -> Bus Creator4/3  "xyh"
  Xe/1 -> xyH1/1  "xyz"
  Bus Creator4/1 -> Aircraft BUS/1  "Aircraft Bus"
  CTRL BUS/1 -> Bus Creator4/8
  AD BUS/1 -> Bus Creator4/9
  PD BUS/1 -> Bus Creator4/10
  ENV BUS/1 -> Bus Creator4/11
  Demux/2 -> Bus Creator/2  "CY"
  Demux/6 -> Bus Creator/6  "Cn"
  Bus Creator/1 -> Bus Creator4/12  "AERO BUS"
  Demux/4 -> Bus Creator/4  "Cl"
  Demux/1 -> Bus Creator/1  "CX"
  Demux/3 -> Bus Creator/3  "CZ"
  AeroCoeff/1 -> Demux/1
  Demux/5 -> Bus Creator/5  "Cm"
  XYZ Total/1 -> Bus Creator4/13  "XYZ Total"

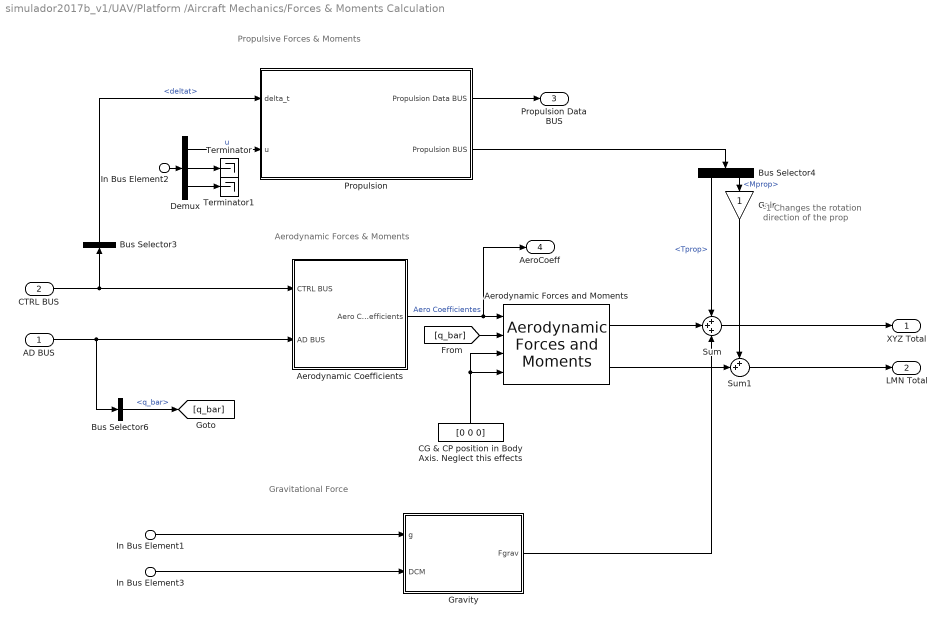
== system simulador2017b_v1/UAV/Platform /Aircraft Mechanics/Forces & Moments Calculation ==
  note: Gravitational Force
  note: Aerodynamic Forces & Moments
  note: Propulsive Forces & Moments
  note: -1 Changes the
      | rotation direction
      | of the prop
  AD BUS : Inport
  CTRL BUS : Inport  Port=2
  In Bus Element2 : Inport  Port=3  PortName=AC BUS  Element=uvw
  In Bus Element3 : Inport  Port=3  PortName=AC BUS  Element=DCMbe
  In Bus Element1 : Inport  Port=4  PortName=ENV BUS  Element=g
  "Aerodynamic Forces and Moments " : aerolibadyn/Aerodynamic Forces and Moments   inputAxes=Body  outputForceAxes=Body  outputMomentAxes=Body  S=S  b=b  cbar=c_bar
      settings: SourceProductName=Aerospace Blockset
  "Aerodynamic Coefficients " : Subsystem
  Bus Selector3 : BusSelector  OutputSignals=deltat
  Bus Selector4 : BusSelector  OutputSignals=Tprop,Mprop
  Bus Selector6 : BusSelector  OutputSignals=q_bar
  CG & CP position in Body Axis. Neglect this effects : Constant  Value=[0 0 0]
  Demux : Demux  Outputs=3
  Gain : Gain
  "Gravity " : Subsystem
      mask Display:
      | port_label('input',1,'g','texmode','on')
      | port_label('input',2,'DCM_e^b','texmode','on')
      | port_label('output',1,'F_g','texmode','on')
  Propulsion : Subsystem
      mask Display:
      | port_label('input',2,'u Front Airflow Velocity','texmode','on')
      | port_label('input',1,'\delta_t Throttle','texmode','on')
      | port_label('output',2,'T_x , Q_x','texmode','on')
      | port_label('output',1,'Propulsion Data BUS (PD BUS)','texmode','on')
  Sum : Sum  Inputs=+++
  Sum1 : Sum  Inputs=++|
  Terminator : Terminator
  Terminator1 : Terminator
  XYZ Total : Outport
  LMN Total : Outport  Port=2
  "Propulsion Data BUS " : Outport  Port=3
  AeroCoeff : Outport  Port=4
  wires:
  "Gravity "/1(Fgrav) -> Sum/3
  Sum/1 -> XYZ Total/1
  "Aerodynamic Forces and Moments "/1 -> Sum/2
  In Bus Element3/1 -> "Gravity "/2(DCM)
  In Bus Element2/1 -> Demux/1
  CTRL BUS/1 -> "Aerodynamic Coefficients "/1(CTRL BUS), Bus Selector3/1
  "Aerodynamic Forces and Moments "/2 -> Sum1/2
  Sum1/1 -> LMN Total/1
  Bus Selector4/1 -> Sum/1  "<Tprop>"
  Propulsion/1(Propulsion Data BUS) -> "Propulsion Data BUS "/1
  Bus Selector4/2 -> Gain/1  "<Mprop>"
  Propulsion/2(Propulsion BUS) -> Bus Selector4/1
  Bus Selector3/1 -> Propulsion/1(delta_t)  "<deltat>"
  Demux/3 -> Terminator1/1
  Demux/2 -> Terminator/1
  Demux/1 -> Propulsion/2(u)  "u"
  Gain/1 -> Sum1/1
  AD BUS/1 -> Bus Selector6/1, "Aerodynamic Coefficients "/2(AD BUS)
  CG & CP position in Body Axis. Neglect this effects/1 -> "Aerodynamic Forces and Moments "/4, "Aerodynamic Forces and Moments "/3
  "Aerodynamic Coefficients "/1("Aero Coefficients ") -> AeroCoeff/1, "Aerodynamic Forces and Moments "/1  "Aero Coefficientes"
  Bus Selector6/1 -> [q_bar]  "<q_bar>"
  In Bus Element1/1 -> "Gravity "/1(g)
  [q_bar] -> "Aerodynamic Forces and Moments "/2

== system simulador2017b_v1/UAV/Platform /Aircraft Mechanics/Forces & Moments Calculation/Aerodynamic Coefficients  ==
  note: The projection could be executed in this segment of the diagram,
      | just before the final sum (it would be a better practice to keep things more clear) .
  note: CL and CD forces are projected in body axis
      | and expressed as Cx and Cz.
      |
      | The projection occurs inside this block
  note: Compute Coefficients
  note: Signal preparation
  CTRL BUS : Inport
  Bus Element In : Inport  Port=2  PortName=AD BUS  Element=alpha
  Bus Element In1 : Inport  Port=2  PortName=AD BUS  Element=beta
  Bus Element In2 : Inport  Port=2  PortName=AD BUS  Element=Va
  Bus Element In3 : Inport  Port=2  PortName=AD BUS  Element=pqr_tot
  Actuator Increments : Subsystem
      mask Display:
      | port_label('input',1,'[\delta_a,\delta_e,\delta_r,\delta_f]','texmode','on')
      | port_label('input',2,'[C_{X_{\delta_e}},C_{Z_{\delta_e}}]','texmode','on')
      | port_label('output',1,'Coefficients','texmode','on')
  Aerodynamic Actuators : Subsystem
      mask Display:
      | port_label('input',1,'CTRL BUS','texmode','on')
      | port_label('output',1,'[\delta_a,\delta_e,\delta_r,\delta_f]','texmode','on')
  Body Rate Damping : Subsystem
      mask Display:
      | port_label('input',1,'V_{aero}','texmode','on')
      | port_label('input',2,'[p,q,r]','texmode','on')
      | port_label('input',3,'[C_{X_q},C_{Z_q}]','texmode','on')
      | port_label('output',1,'Coefficients','texmode','on')
  Bus Selector : BusSelector  OutputSignals=qCoef
  Bus Selector3 : BusSelector  OutputSignals=deltaeCoef
  Bus Selector4 : BusSelector  OutputSignals=alphaFunctions
  "Longitudinal Aerodynamics (Cx, Cz, Cm coefficients)" : Subsystem
      mask Display: image('C:\Users\rablanco.ext\Desktop\lognitudinal aerodynamics.png');
  Sum : Sum  Inputs=+++  SaturateOnIntegerOverflow=on
  alpha-beta Coefficients : Subsystem
      mask Display:
      | port_label('input',1,'\beta','texmode','on')
      | port_label('input',2,'C_X(\alpha), C_Z(\alpha), C_m(\alpha)','texmode','on')
      | port_label('output',1,'Coefficients','texmode','on')
  "Aero Coefficients " : Outport
  wires:
  "Longitudinal Aerodynamics (Cx, Cz, Cm coefficients)"/1(CX,CZ,Cm) -> Bus Selector/1, Bus Selector3/1, Bus Selector4/1  "Long Aero Coef BUS"
  Bus Element In/1 -> "Longitudinal Aerodynamics (Cx, Cz, Cm coefficients)"/1("alpha ")  "alpha"
  alpha-beta Coefficients/1(Coefficients) -> Sum/1
  Body Rate Damping/1(Coefficients) -> Sum/3
  Actuator Increments/1(Coefficients) -> Sum/2
  Bus Element In1/1 -> alpha-beta Coefficients/1(beta)
  Sum/1 -> "Aero Coefficients "/1
  Bus Element In3/1 -> Body Rate Damping/2(p,q,r)
  Bus Element In2/1 -> Body Rate Damping/1(V)
  CTRL BUS/1 -> Aerodynamic Actuators/1(CTRL BUS)
  Aerodynamic Actuators/1(Surface Signals) -> Actuator Increments/1(Actuator Deflections)
  Bus Selector3/1 -> Actuator Increments/2(deltaeCoef)  "<deltaeCoef>"
  Bus Selector/1 -> Body Rate Damping/3("qCoef ")  "<qCoef>"
  Bus Selector4/1 -> alpha-beta Coefficients/2(Longitudinal Aerodynamics)  "<alphaFunctions>"

== system simulador2017b_v1/UAV/Platform /Aircraft Mechanics/Forces & Moments Calculation/Gravity  ==
  g : Inport  Unit=m/s^2
  DCM : Inport  Port=2
  Gravity in Earth Axes : Gain  Gain=mass  SaturateOnIntegerOverflow=on  OutDataTypeStr=Inherit: Same as input  ParamDataTypeStr=Inherit: Same as input
  Inertial to Body : Product  Multiplication=Matrix(*)  SaturateOnIntegerOverflow=on  InputSameDT=on  OutDataTypeStr=Inherit: Same as first input
  Fgrav : Outport  Unit=N
  wires:
  DCM/1 -> Inertial to Body/1
  g/1 -> Gravity in Earth Axes/1
  Inertial to Body/1 -> Fgrav/1
  Gravity in Earth Axes/1 -> Inertial to Body/2

== system simulador2017b_v1/UAV/Platform /Aircraft Mechanics/Forces & Moments Calculation/Propulsion ==
  note: Algebraic Loop (Torque)
  delta_t : Inport
  u : Inport  Port=2
  1 dim to 6 dim1 : Subsystem
  Bus Creator1 : BusCreator  Inputs=3
  Motor : Subsystem
  Propeller : Subsystem
  Propulsion Data BUS : Outport
  Propulsion BUS : Outport  Port=2
  wires:
  u/1 -> Propeller/2(u)  "u"
  Propeller/1(Tprop) -> 1 dim to 6 dim1/1(Tprop), Bus Creator1/2  "Thrust"
  Propeller/2(Qprop) -> Motor/2(Torque), 1 dim to 6 dim1/2(Qprop), Bus Creator1/3  "Torque"
  Bus Creator1/1 -> Propulsion Data BUS/1  "Propulsion Data BUS"
  1 dim to 6 dim1/1(Propulsion BUS) -> Propulsion BUS/1
  Motor/1(RPM) -> Propeller/1(RPM), Bus Creator1/1  "RPM"
  delta_t/1 -> Motor/1(Throttle)  "Throttle"
